simulink model "Sim_main"  (R2025a)
settings: Solver=FixedStepAuto  StartTime=0.0  StopTime=8760  FixedStep=1  RelTol=1e-3
values from neighbouring files (symbols this model uses):
  A = R * 2 * H    [LCOW_calculation.m]    (also in RUN_Simulink_POOL.m; RUN_Simulink_RandomSet.m; RUN_Simulink_SINGLE.m = 12.786871552)
  Cf = 36000    [RUN_Simulink_POOL.m]    (also in RUN_Simulink_RandomSet.m; RUN_Simulink_SINGLE.m)
  CutIn = 3    [RUN_Simulink_POOL.m]    (also in RUN_Simulink_RandomSet.m; RUN_Simulink_SINGLE.m)
  IP1 = (n/(n-1))*P1*( (P2/P1)^((n-1)/n) - 1)    (= 259255.992944)    [RUN_Simulink_POOL.m]    (also in RUN_Simulink_RandomSet.m; RUN_Simulink_SINGLE.m)
  J1 = 1.5 * As    [RUN_Simulink_POOL.m]    (also in RUN_Simulink_RandomSet.m; RUN_Simulink_SINGLE.m = 4.38)
  Limit_Tor = Tor_rq * 0.5    (= 2.3371585434)    [RUN_Simulink_POOL.m]    (also in RUN_Simulink_RandomSet.m; RUN_Simulink_SINGLE.m = 3.45899464424)
  N_PV = data.N_PV(i)    [LCOW_calculation.m]    (also in MOO_Qp_LCOW_CO2.m = optimvar("N_PV","Type","integer","LowerBound",1,"UpperBound"; RUN_Simulink_POOL.m = N_PV_values(i); RUN_Simulink_RandomSet.m = N_PV_values; RUN_Simulink_SINGLE.m = 2)
  N_ro = data.N_ro(i)    [LCOW_calculation.m]    (also in MOO_Qp_LCOW_CO2.m = optimvar("N_ro","Type","integer","LowerBound",2,"UpperBound"; RUN_Simulink_POOL.m = N_ro_values(i); RUN_Simulink_RandomSet.m = N_ro_values; RUN_Simulink_SINGLE.m = 6)
  Nt = data.Nt(i)    [LCOW_calculation.m]    (also in MOO_Qp_LCOW_CO2.m = optimvar("Nt","Type","integer","LowerBound",10,"UpperBound",; RUN_Simulink_POOL.m = Nt_values(i); RUN_Simulink_RandomSet.m = Nt_values; RUN_Simulink_SINGLE.m = 58)
  P2 = 800000    [RUN_Simulink_POOL.m]    (also in RUN_Simulink_RandomSet.m; RUN_Simulink_SINGLE.m)
  R = 0.515 * As    [LCOW_calculation.m]    (also in RUN_Simulink_POOL.m; RUN_Simulink_RandomSet.m; RUN_Simulink_SINGLE.m = 1.5038)
  Tor_rq = IP1 * Va * 10 / (17 * pi)    (= 4.67431708681)    [RUN_Simulink_POOL.m]    (also in RUN_Simulink_RandomSet.m; RUN_Simulink_SINGLE.m = 6.91798928848)
  TR = data.TR(i)    [LCOW_calculation.m]    (also in MOO_Qp_LCOW_CO2.m = optimvar("TR","LowerBound",3,"UpperBound",10); RUN_Simulink_POOL.m = TR_values(i); RUN_Simulink_RandomSet.m = TR_values; RUN_Simulink_SINGLE.m = 9.36)
  Va = e_vol * Vs    (= 9.6291546017e-05)    [RUN_Simulink_POOL.m]    (also in RUN_Simulink_RandomSet.m; RUN_Simulink_SINGLE.m = 0.000142511488105)
  Vf1 = ((P1+Pa)*T2/(T1*(P2+Pa)))*1000    (= 339.891157105)    [RUN_Simulink_POOL.m]    (also in RUN_Simulink_RandomSet.m; RUN_Simulink_SINGLE.m)
  Vt = 2000    [RUN_Simulink_POOL.m]    (also in RUN_Simulink_RandomSet.m; RUN_Simulink_SINGLE.m)
undefined symbols (not defined in the file or in its folder): magnitude
libraries: statsLibrary x36, simulink x1
(part 3 of 4)

== system Sim_main/Transmission ==
  note: Transmission ratios and lossws on the system
  note: Q_pump = Q_rotor (1- losses_trans )*i
  note: W_pump = W_rotor*i
  note: Transmission ratios of rotaional speed
  W_rotor : Inport
  Torque : Inport  Port=2
  Divide : Product  Inputs=/*  RndMeth=Zero  SaturateOnIntegerOverflow=on
  Product : Product
  losses_trans : Gain  Gain=1-0.12
  trans_ratio : Constant  Value=TR
  trans_ratio1 : Constant  Value=TR
  W_Trans : Outport
  Q_trans : Outport  Port=2
  wires:
  trans_ratio1/1 -> Divide/1
  Divide/1 -> losses_trans/1
  losses_trans/1 -> Q_trans/1
  W_rotor/1 -> Product/2
  Torque/1 -> Divide/2
  trans_ratio/1 -> Product/1
  Product/1 -> W_Trans/1

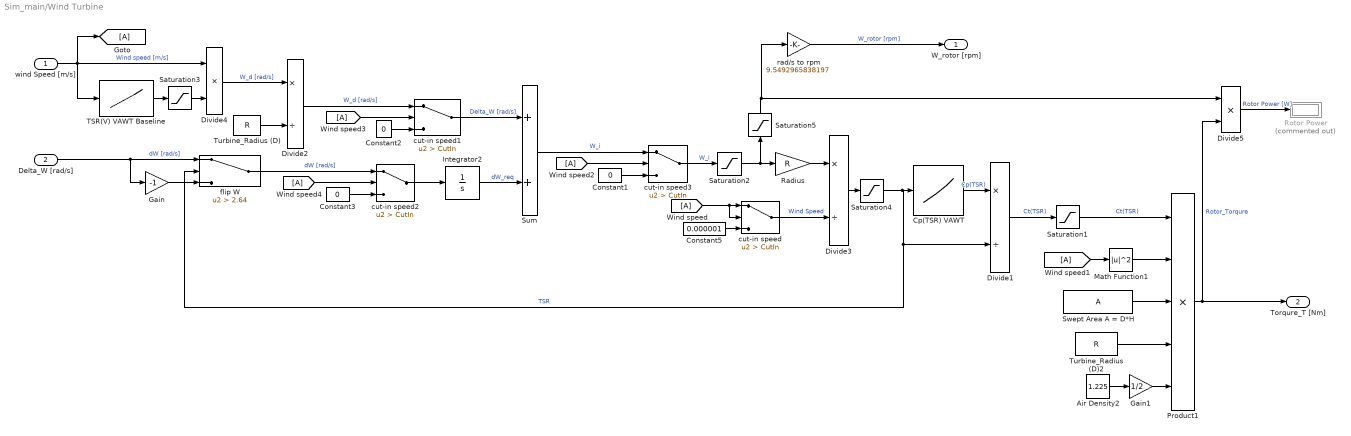
== system Sim_main/Wind Turbine ==
  wind Speed [m/s] : Inport
  Delta_W [rad/s] : Inport  Port=2
  Air Density2 : Constant  Value=1.225
  Constant1 : Constant  Value=0
  Constant2 : Constant  Value=0
  Constant3 : Constant  Value=0
  Constant5 : Constant  Value=0.000001
  Cp(TSR) VAWT : Lookup_n-D  NumberOfTableDimensions=1  BreakpointsForDimension1=[1.439502;1.679111;2.035892;2.329388;2.509915;2.636906;3.080976;3.291367]  Table=[0.01305;0.045283;0.137264;0.259906;0.301179;0.312972;0.285063;0.25283]  InternalRulePriority=Speed  RndMeth=Simplest
  Divide1 : Product  Inputs=*/
  Divide2 : Product  Inputs=*/
  Divide3 : Product  Inputs=*/
  Divide4 : Product  Inputs=**
  Divide5 : Product  Inputs=**
  Gain : Gain  Gain=-1
  Gain1 : Gain  Gain=1/2
  Goto : Goto
  Integrator2 : Integrator  LowerSaturationLimit=-3
  Math Function1 : Math  Operator=magnitude^2
  Product1 : Product  Inputs=5
  Radius : Gain  Gain=R
  Rotor Power : Display  Commented=on
  Saturation1 : Saturate  UpperLimit=inf  LowerLimit=0
  Saturation2 : Saturate  UpperLimit=inf  LowerLimit=0
  Saturation3 : Saturate  UpperLimit=inf  LowerLimit=0.000001
  Saturation4 : Saturate  UpperLimit=6  LowerLimit=0.000001
  Saturation5 : Saturate  UpperLimit=inf  LowerLimit=0.000001
  Sum : Sum
  Swept Area A = D*H : Constant  Value=A
  TSR(V) VAWT Baseline : Lookup_n-D  NumberOfTableDimensions=1  BreakpointsForDimension1=[1;2;4;6;8;10;12]  Table=[0;1;2.4;2.85;3.57;3.96;4.22]  InternalRulePriority=Speed  RndMeth=Simplest
  Turbine_Radius (D) : Constant  Value=R
  Turbine_Radius (D)2 : Constant  Value=R
  Wind speed{,1..4} (5 alike) : From
  cut-in speed{,1..3} (4 alike) : Switch  Criteria=u2 > Threshold  Threshold=CutIn  SaturateOnIntegerOverflow=off  InputSameDT=off
  flip W : Switch  Criteria=u2 > Threshold  Threshold=2.64  SaturateOnIntegerOverflow=off  InputSameDT=off
  rad/s to rpm : Gain  Gain=9.5492965838197
  W_rotor [rpm] : Outport
  Torqure_T [Nm] : Outport  Port=2
  wires:
  wind Speed [m/s]/1 -> Goto/1, TSR(V) VAWT Baseline/1, Divide4/1  "Wind speed [m/s]"
  Divide5/1 -> Rotor Power/1  "Rotor Power [W]"
  Wind speed4/1 -> cut-in speed2/2
  Divide4/1 -> Divide2/1  "W_d [rad/s]"
  Saturation3/1 -> Divide4/2
  TSR(V) VAWT Baseline/1 -> Saturation3/1
  Sum/1 -> cut-in speed3/1  "W_i"
  Wind speed2/1 -> cut-in speed3/2
  Constant1/1 -> cut-in speed3/3
  cut-in speed2/1 -> Integrator2/1
  cut-in speed/1 -> Divide3/2  "Wind Speed"
  Constant5/1 -> cut-in speed/3
  Wind speed/1 -> cut-in speed/2, cut-in speed/1
  Constant3/1 -> cut-in speed2/3
  cut-in speed1/1 -> Sum/1  "Delta_W [rad/s]"
  Constant2/1 -> cut-in speed1/3
  Wind speed3/1 -> cut-in speed1/2
  rad/s to rpm/1 -> W_rotor [rpm]/1  "W_rotor [rpm]"
  Saturation1/1 -> Product1/1  "Ct(TSR)"
  Cp(TSR) VAWT/1 -> Divide1/1  "Cp(TSR)"
  Gain1/1 -> Product1/5
  Divide2/1 -> cut-in speed1/1  "W_d [rad/s]"
  Product1/1 -> Torqure_T [Nm]/1, Divide5/2  "Rotor_Torqure"
  Turbine_Radius (D)2/1 -> Product1/4
  Swept Area A = D*H/1 -> Product1/3
  Wind speed1/1 -> Math Function1/1
  Math Function1/1 -> Product1/2
  Air Density2/1 -> Gain1/1
  Divide1/1 -> Saturation1/1  "Ct(TSR)"
  Divide3/1 -> Saturation4/1
  Radius/1 -> Divide3/1
  Turbine_Radius (D)/1 -> Divide2/2
  cut-in speed3/1 -> Saturation2/1  "W_i"
  Saturation2/1 -> Saturation5/1, Radius/1
  Saturation5/1 -> rad/s to rpm/1, Divide5/1
  Integrator2/1 -> Sum/2  "dW_req"
  flip W/1 -> cut-in speed2/1  "dW [rad/s]"
  Gain/1 -> flip W/3
  Delta_W [rad/s]/1 -> Gain/1, flip W/1  "dW [rad/s]"
  Saturation4/1 -> flip W/2, Divide1/2, Cp(TSR) VAWT/1  "TSR"

== system Sim_main/Pumps/Air operated pump ==
  Air_in : Inport
  P_in : Inport  Port=2
  Air [l/s] to water buckup1 : Lookup_n-D  BreakpointsForDimension1=[1;4;6;8;10;12;14]  BreakpointsForDimension2=[4.8 6.8 8.3]  Table=[6.4 4.22 3.7;28.27 20.5 17.54;44.82 32.5 27.24;63.58 45.5 34.6;86.46 59.3 49;86.46 75.2 61.37;86.46 93 73.8]  InternalRulePriority=Speed  RndMeth=Simplest
      settings: InputPortMap=u0,u1
  Gain1 : Gain  Gain=1/3600
  Saturation : Saturate  UpperLimit=inf  LowerLimit=0
  Saturation2 : Saturate  UpperLimit=inf  LowerLimit=0
  buckup1 : Lookup_n-D  BreakpointsForDimension1=[1;2.76;4.52;6.28;8.04;9.8;11.56;13.32;15.08;16.84;18.6;20.36;22.12;23.88;25.64;27.4;29.16;30.92;32.68;34.44;36.2;37.96;39.72;41.48;43.24;45;46.76;48.52;50.28;52.04;53.8;55.56;57.32;59.08;60.84;62.6;64.36;66.12;67.88;69.64;71.4;73.16;74.92;76.68;78.44;80.2]  BreakpointsForDimension2=[4.8;6.8;8.3]  Table=[33.96748 49.87303 59.5914;33.76481 49.31838 58.97968;33.48128 48.77087 58.35368;33.14781 48.22336 57.75622;32.88569 47.71152 57.1445;32.55935 47.18541 56.49234;32.26869 46.66644 56.03308;31.94236 46.14746 55.45677;31.65883 45.63562 54.78321;31.32536 45.15232 54.24284;31.02043 44.63335 53.65252;30.7155 44.13578 53.0836;30.39629 43.67389 52.53609;30.0985 43.21199 51.96717;29.76503 42.70015 51.41252;29.46723 42.25966 50.85074;29.14089 41.79063 50.32463;28.81456 41.31446 49.78425;28.50249 40.8597 49.23674;28.15475 40.42634 48.71777;27.84982 39.95731 48.19879;27.53062 39.54536 47.68695;27.21142 39.112 47.17511;26.90649 38.68578 46.65614;26.54448 38.25956 46.1443;26.21814 37.8048 45.64673;25.89181 37.58073 45.14203;25.55834 37.04273 44.673;25.21773 36.65456 44.20397;24.90567 36.26401 43.71353;24.53652 35.8806 43.2231;24.21732 35.45913 42.71601;23.86958 35.11377 42.31357;23.52898 34.7803 41.88735;23.18837 34.41829 41.36124;22.84776 34.05628 40.91362;22.50003 33.69427 40.44459;22.15942 33.3394 40.08258;21.81881 33.00593 39.63495;21.45681 32.62965 39.19446;21.10907 32.36752 38.7611;20.77559 32.02692 38.27542;20.40645 31.70058 37.82304;20.05871 31.38852 37.62751;19.70384 31.07645 37.26074;19.22529 30.84559 36.75502]  InternalRulePriority=Speed  RndMeth=Simplest
      settings: InputPortMap=u0,u1
  l/m to m3/h : Gain  Gain=0.06
  Feed flow m3/h : Outport
  Backpressure [bar] : Outport  Port=2
  wires:
  l/m to m3/h/1 -> Feed flow m3/h/1  "Feed flow m3/h"
  Air [l/s] to water buckup1/1 -> Saturation2/1  "water L/m"
  Air_in/1 -> Gain1/1
  Gain1/1 -> Air [l/s] to water buckup1/1
  P_in/1 -> Air [l/s] to water buckup1/2, buckup1/2
  buckup1/1 -> Saturation/1
  Saturation/1 -> Backpressure [bar]/1
  Saturation2/1 -> buckup1/1, l/m to m3/h/1

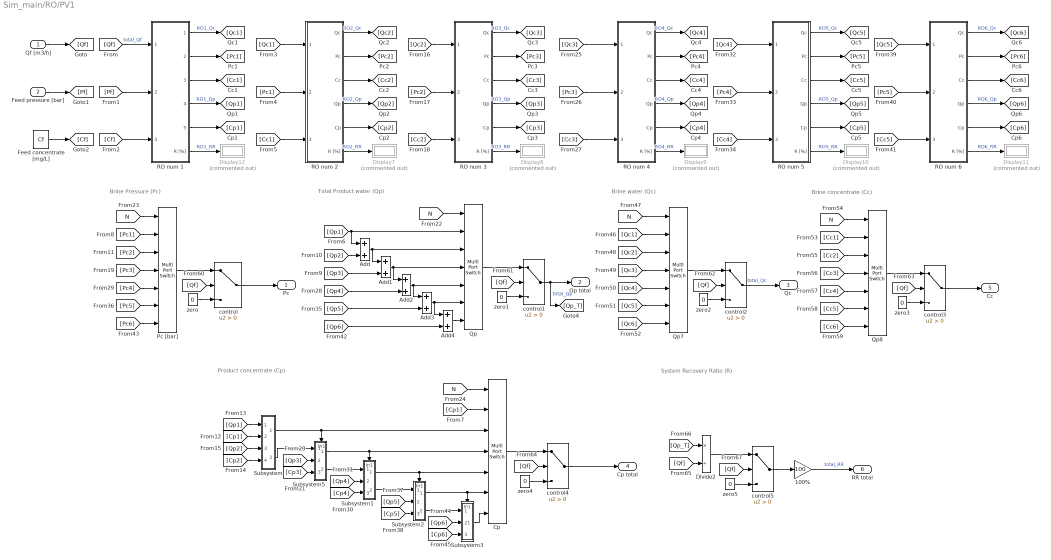
== system Sim_main/RO/PV1 ==
  note: System Recovery Ratio (R)
  note: Brine concentrate (Cc)
  note: Product concentrate (Cp)
  note: Brine water (Qc)
  note: Total Product water (Qp)
  note: Brine Pressure (Pc)
  Qf [m3/h] : Inport
  Feed pressure [bar] : Inport  Port=2
  100% : Gain  Gain=100
  Add{,1..4} (5 alike) : Sum
  Cp : MultiPortSwitch  Inputs=6  SaturateOnIntegerOverflow=off  InputSameDT=off
  Display{7..12} (6 alike) : Display  Commented=on
  Divide2 : Product  Inputs=*/
  Feed concentrate [mg/L] : Constant  Value=Cf
  Pc [bar] : MultiPortSwitch  Inputs=6  SaturateOnIntegerOverflow=off  InputSameDT=off
  Qp : MultiPortSwitch  Inputs=6  SaturateOnIntegerOverflow=off  InputSameDT=off
  Qp7 : MultiPortSwitch  Inputs=6  SaturateOnIntegerOverflow=off  InputSameDT=off
  Qp8 : MultiPortSwitch  Inputs=6  SaturateOnIntegerOverflow=off  InputSameDT=off
  RO num 1 : Subsystem
  RO num 2 : Subsystem
  RO num 3 : Subsystem
  RO num 4 : Subsystem
  RO num 5 : Subsystem
  RO num 6 : Subsystem
  Subsystem : Subsystem
  Subsystem1 : Subsystem
      settings: PortSchema="{\"entries\":[{\"content\":{\"sides\":[{\"content\":{\"connectorIds\":[\"In1\",\"In2\",\"In3\"]},\"type\":\"ConnectorPlacement.EquallySpacedRectSide\",\"uuid\":\"d5ba013f-6078-4f30-8328-72ed2cb8129b\"},{\"content\":{\"connectorIds\":[\"Out1\",\"Out2\"],\"side\":\"RIGHT\"},\"type\":\"ConnectorPlacement.EquallySpacedRectSide\",\"uuid\":\"ed7cb065-416c-47c0-a617-1717dea4ab53\"},{\"content\":{\"connectorIds\":[\"In4\"],\"side\":\"TOP\"},\"type\":\"ConnectorPlacement.EquallySpacedRectSide\",\"uuid\":\"ec2d37e4-f712-4138-a382-b2b31ae58dd4\"}]},\"type\":\"ConnectorPlacement.EquallySpacedConnector\",\"uuid\":\"e33a2c60-ddf6-4c9a-9e3a-37228ac662ce\"}],\"packageUris\":[\"http://schema.mathworks.com/mf0/Connector/R2020b\"],\"version\":\"1.0\"}"
  Subsystem2 : Subsystem
      settings: PortSchema="{\"entries\":[{\"content\":{\"sides\":[{\"content\":{\"connectorIds\":[\"In1\",\"In2\",\"In3\"]},\"type\":\"ConnectorPlacement.EquallySpacedRectSide\",\"uuid\":\"d5ba013f-6078-4f30-8328-72ed2cb8129b\"},{\"content\":{\"connectorIds\":[\"Out1\",\"Out2\"],\"side\":\"RIGHT\"},\"type\":\"ConnectorPlacement.EquallySpacedRectSide\",\"uuid\":\"ed7cb065-416c-47c0-a617-1717dea4ab53\"},{\"content\":{\"connectorIds\":[\"In4\"],\"side\":\"TOP\"},\"type\":\"ConnectorPlacement.EquallySpacedRectSide\",\"uuid\":\"ec2d37e4-f712-4138-a382-b2b31ae58dd4\"}]},\"type\":\"ConnectorPlacement.EquallySpacedConnector\",\"uuid\":\"e33a2c60-ddf6-4c9a-9e3a-37228ac662ce\"}],\"packageUris\":[\"http://schema.mathworks.com/mf0/Connector/R2020b\"],\"version\":\"1.0\"}"
  Subsystem3 : Subsystem
      settings: PortSchema="{\"entries\":[{\"content\":{\"sides\":[{\"content\":{\"connectorIds\":[\"In1\",\"In2\",\"In3\"]},\"type\":\"ConnectorPlacement.EquallySpacedRectSide\",\"uuid\":\"d5ba013f-6078-4f30-8328-72ed2cb8129b\"},{\"content\":{\"connectorIds\":[\"Out1\"],\"side\":\"RIGHT\"},\"type\":\"ConnectorPlacement.EquallySpacedRectSide\",\"uuid\":\"ed7cb065-416c-47c0-a617-1717dea4ab53\"},{\"content\":{\"connectorIds\":[\"In4\"],\"side\":\"TOP\"},\"type\":\"ConnectorPlacement.EquallySpacedRectSide\",\"uuid\":\"ec2d37e4-f712-4138-a382-b2b31ae58dd4\"}]},\"type\":\"ConnectorPlacement.EquallySpacedConnector\",\"uuid\":\"e33a2c60-ddf6-4c9a-9e3a-37228ac662ce\"}],\"packageUris\":[\"http://schema.mathworks.com/mf0/Connector/R2020b\"],\"version\":\"1.0\"}"
  Subsystem5 : Subsystem
      settings: PortSchema="{\"entries\":[{\"content\":{\"sides\":[{\"content\":{\"connectorIds\":[\"In1\",\"In2\",\"In3\"]},\"type\":\"ConnectorPlacement.EquallySpacedRectSide\",\"uuid\":\"d5ba013f-6078-4f30-8328-72ed2cb8129b\"},{\"content\":{\"connectorIds\":[\"Out1\",\"Out2\"],\"side\":\"RIGHT\"},\"type\":\"ConnectorPlacement.EquallySpacedRectSide\",\"uuid\":\"ed7cb065-416c-47c0-a617-1717dea4ab53\"},{\"content\":{\"connectorIds\":[\"In4\"],\"side\":\"TOP\"},\"type\":\"ConnectorPlacement.EquallySpacedRectSide\",\"uuid\":\"ec2d37e4-f712-4138-a382-b2b31ae58dd4\"}]},\"type\":\"ConnectorPlacement.EquallySpacedConnector\",\"uuid\":\"e33a2c60-ddf6-4c9a-9e3a-37228ac662ce\"}],\"packageUris\":[\"http://schema.mathworks.com/mf0/Connector/R2020b\"],\"version\":\"1.0\"}"
  control{,1..5} (6 alike) : Switch  Criteria=u2 > Threshold  ZeroCross=off  SaturateOnIntegerOverflow=off  InputSameDT=off
  zero{,1..5} (6 alike) : Constant  Value=0
  Pc : Outport
  Qp total : Outport  Port=2
  Qc : Outport  Port=3
  Cp total : Outport  Port=4
  Cc : Outport  Port=5
  RR total : Outport  Port=6
  wires:
  RO num 1/6(R [%]) -> Display12/1  "RO1_RR"
  Add3/1 -> Add4/1, Qp/6
  [Cp1] -> Subsystem/2(In2)
  [Qp4] -> Add2/2
  RO num 5/1(Qc) -> [Qc5]  "RO5_Qc"
  Subsystem/2(Out2) -> Subsystem5/1(In2)
  [Qp4] -> Subsystem1/2(In3)
  RO num 6/5(Cp) -> [Cp6]
  [Pc1] -> Pc [bar]/2
  zero/1 -> control/3
  Subsystem3/1(Out1) -> Cp/7
  [Cc1] -> Qp8/2
  Qp7/1 -> control2/1
  [Qp2] -> Add/2
  [Pf] -> RO num 1/2(Pf [bar])
  [Qc4] -> RO num 5/1(Qf [m3/h])
  Add/1 -> Qp/3, Add1/1
  control1/1 -> Qp total/1, [Qp_T]  "total_Qp"
  RO num 4/2(Pc) -> [Pc4]
  Qf [m3/h]/1 -> [Qf]
  [Cc2] -> Qp8/3
  Qp/1 -> control1/1
  RO num 3/4(Qp) -> [Qp3]  "RO3_Qp"
  [Cp4] -> Subsystem1/3(In4)
  [Pc2] -> RO num 3/2(Pf [bar])
  [Cc5] -> RO num 6/3(Cf [mg/L])
  RO num 6/6(R [%]) -> Display11/1  "RO6_RR"
  [Qp2] -> Subsystem/3(In3)
  [Qc5] -> Qp7/6
  [N] -> Qp8/1
  [Qf] -> control4/2
  RO num 5/6(R [%]) -> Display10/1  "RO5_RR"
  [Qp3] -> Add1/2
  [Qp1] -> Add/1, Qp/2
  RO num 2/3(Cc) -> [Cc2]
  Subsystem2/1(Out1) -> Cp/6, Subsystem3/4(In1)
  Add1/1 -> Qp/4, Add2/1
  RO num 4/5(Cp) -> [Cp4]
  RO num 3/2(Pc) -> [Pc3]
  [Pc2] -> Pc [bar]/3
  RO num 5/2(Pc) -> [Pc5]
  [Pc5] -> Pc [bar]/6
  Add4/1 -> Qp/7
  Feed pressure [bar]/1 -> [Pf]
  RO num 3/1(Qc) -> [Qc3]  "RO3_Qc"
  RO num 6/4(Qp) -> [Qp6]  "RO6_Qp"
  RO num 6/2(Pc) -> [Pc6]
  [Qc3] -> Qp7/4
  Subsystem2/2(Out2) -> Subsystem3/1(In2)
  RO num 5/4(Qp) -> [Qp5]  "RO5_Qp"
  [Cp6] -> Subsystem3/3(In4)
  RO num 1/2(Pc [bar]) -> [Pc1]
  [N] -> Qp7/1
  100%/1 -> RR total/1  "total_RR"
  [Qf] -> control2/2
  Cp/1 -> control4/1
  Subsystem/1(Out1) -> Subsystem5/4(In1), Cp/3
  [Qc5] -> RO num 6/1(Qf [m3/h])
  [Qp5] -> Subsystem2/2(In3)
  RO num 4/1(Qc) -> [Qc4]  "RO4_Qc"
  RO num 1/3(TDSc [mg/L]) -> [Cc1]
  RO num 4/3(Cc) -> [Cc4]
  RO num 2/6(R [%]) -> Display7/1  "RO2_RR"
  RO num 4/6(R [%]) -> Display9/1  "RO4_RR"
  Subsystem5/2(Out2) -> Subsystem1/1(In2)
  control2/1 -> Qc/1  "total_Qc"
  RO num 6/1(Qc) -> [Qc6]  "RO6_Qc"
  [Qp1] -> Subsystem/1(In1)
  [Cc6] -> Qp8/7
  [Cf] -> RO num 1/3(TDSf [mg/L])
  [N] -> Cp/1
  [Cc4] -> Qp8/5
  [Pc4] -> Pc [bar]/5
  RO num 2/2(Pc) -> [Pc2]
  [Qp6] -> Subsystem3/2(In3)
  [Qc3] -> RO num 4/1(Qf [m3/h])
  [Qf] -> RO num 1/1(Qf [m3/h])  "total_Qf"
  [N] -> Qp/1
  Subsystem1/1(Out1) -> Subsystem2/4(In1), Cp/5
  Feed concentrate [mg/L]/1 -> [Cf]
  RO num 1/5(TDSp [mg/L]) -> [Cp1]
  RO num 3/3(Cc) -> [Cc3]
  RO num 1/4(Qp [m3/h]) -> [Qp1]  "RO1_Qp"
  control3/1 -> Cc/1
  [Cc2] -> RO num 3/3(Cf [mg/L])
  RO num 3/5(Cp) -> [Cp3]
  zero5/1 -> control5/3
  [Qp5] -> Add3/2
  Subsystem5/1(Out1) -> Subsystem1/4(In1), Cp/4
  RO num 5/5(Cp) -> [Cp5]
  zero3/1 -> control3/3
  [Qf] -> control/2
  RO num 2/4(Qp) -> [Qp2]  "RO2_Qp"
  [Cp2] -> Subsystem/4(In4)
  [Qp_T] -> Divide2/1
  [Qp3] -> Subsystem5/2(In3)
  [Cp1] -> Cp/2
  Pc [bar]/1 -> control/1
  Divide2/1 -> control5/1
  [Qc6] -> Qp7/7
  [Qp6] -> Add4/2
  [Cc5] -> Qp8/6
  zero4/1 -> control4/3
  [Cc3] -> RO num 4/3(Cf [mg/L])
  zero1/1 -> control1/3
  [Pc3] -> Pc [bar]/4
  [Pc6] -> Pc [bar]/7
  RO num 5/3(Cc) -> [Cc5]
  [Cp5] -> Subsystem2/3(In4)
  [Qf] -> control5/2
  control4/1 -> Cp total/1
  RO num 2/1(Qc) -> [Qc2]  "RO2_Qc"
  [Qf] -> control1/2
  [Qf] -> Divide2/2
  [Cp3] -> Subsystem5/3(In4)
  [Qc2] -> RO num 3/1(Qf [m3/h])
  zero2/1 -> control2/3
  [Pc1] -> RO num 2/2(Pf [bar])
  RO num 4/4(Qp) -> [Qp4]  "RO4_Qp"
  [Cc4] -> RO num 5/3(Cf [mg/L])
  [Qc1] -> Qp7/2
  [Pc3] -> RO num 4/2(Pf [bar])
  RO num 3/6(R [%]) -> Display8/1  "RO3_RR"
  RO num 2/5(Cp) -> [Cp2]
  [Qc4] -> Qp7/5
  Qp8/1 -> control3/1
  [Cc1] -> RO num 2/3(Cf [mg/L])
  [Qc2] -> Qp7/3
  control5/1 -> 100%/1
  [Qf] -> control3/2
  [Pc4] -> RO num 5/2(Pf [bar])
  RO num 6/3(Cc) -> [Cc6]
  Subsystem1/2(Out2) -> Subsystem2/1(In2)
  [Qc1] -> RO num 2/1(Qf [m3/h])
  control/1 -> Pc/1
  Add2/1 -> Qp/5, Add3/1
  [Cc3] -> Qp8/4
  [N] -> Pc [bar]/1
  RO num 1/1(Qc [m3/h]) -> [Qc1]  "RO1_Qc"
  [Pc5] -> RO num 6/2(Pf [bar])

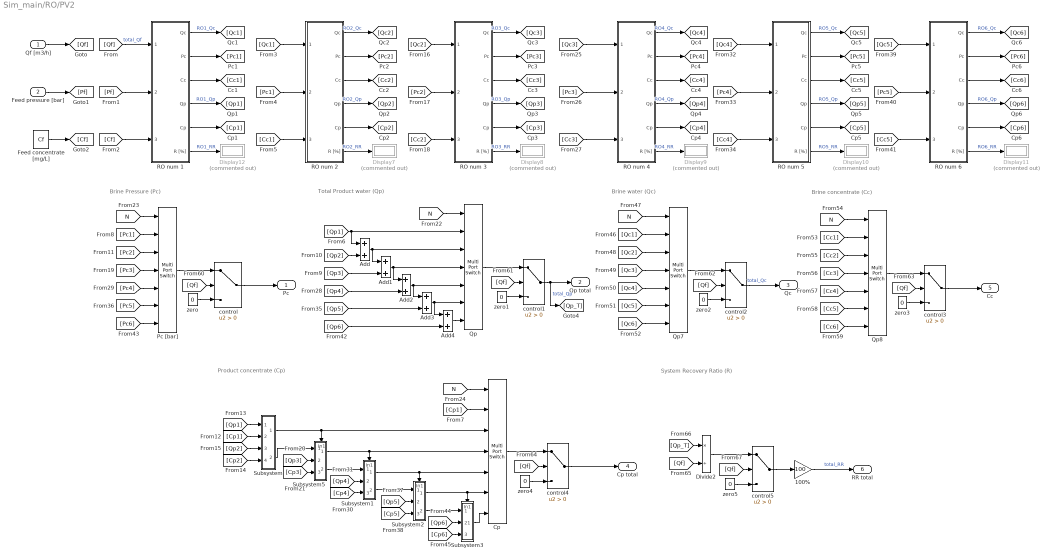
== system Sim_main/RO/PV2 ==
  note: System Recovery Ratio (R)
  note: Brine concentrate (Cc)
  note: Product concentrate (Cp)
  note: Brine water (Qc)
  note: Total Product water (Qp)
  note: Brine Pressure (Pc)
  Qf [m3/h] : Inport
  Feed pressure [bar] : Inport  Port=2
  100% : Gain  Gain=100
  Add{,1..4} (5 alike) : Sum
  Cp : MultiPortSwitch  Inputs=6  SaturateOnIntegerOverflow=off  InputSameDT=off
  Display{7..12} (6 alike) : Display  Commented=on
  Divide2 : Product  Inputs=*/
  Feed concentrate [mg/L] : Constant  Value=Cf
  Pc [bar] : MultiPortSwitch  Inputs=6  SaturateOnIntegerOverflow=off  InputSameDT=off
  Qp : MultiPortSwitch  Inputs=6  SaturateOnIntegerOverflow=off  InputSameDT=off
  Qp7 : MultiPortSwitch  Inputs=6  SaturateOnIntegerOverflow=off  InputSameDT=off
  Qp8 : MultiPortSwitch  Inputs=6  SaturateOnIntegerOverflow=off  InputSameDT=off
  RO num 1 : Subsystem
  RO num 2 : Subsystem
  RO num 3 : Subsystem
  RO num 4 : Subsystem
  RO num 5 : Subsystem
  RO num 6 : Subsystem
  Subsystem : Subsystem
  Subsystem1 : Subsystem
      settings: PortSchema="{\"entries\":[{\"content\":{\"sides\":[{\"content\":{\"connectorIds\":[\"In1\",\"In2\",\"In3\"]},\"type\":\"ConnectorPlacement.EquallySpacedRectSide\",\"uuid\":\"d5ba013f-6078-4f30-8328-72ed2cb8129b\"},{\"content\":{\"connectorIds\":[\"Out1\",\"Out2\"],\"side\":\"RIGHT\"},\"type\":\"ConnectorPlacement.EquallySpacedRectSide\",\"uuid\":\"ed7cb065-416c-47c0-a617-1717dea4ab53\"},{\"content\":{\"connectorIds\":[\"In4\"],\"side\":\"TOP\"},\"type\":\"ConnectorPlacement.EquallySpacedRectSide\",\"uuid\":\"ec2d37e4-f712-4138-a382-b2b31ae58dd4\"}]},\"type\":\"ConnectorPlacement.EquallySpacedConnector\",\"uuid\":\"e33a2c60-ddf6-4c9a-9e3a-37228ac662ce\"}],\"packageUris\":[\"http://schema.mathworks.com/mf0/Connector/R2020b\"],\"version\":\"1.0\"}"
  Subsystem2 : Subsystem
      settings: PortSchema="{\"entries\":[{\"content\":{\"sides\":[{\"content\":{\"connectorIds\":[\"In1\",\"In2\",\"In3\"]},\"type\":\"ConnectorPlacement.EquallySpacedRectSide\",\"uuid\":\"d5ba013f-6078-4f30-8328-72ed2cb8129b\"},{\"content\":{\"connectorIds\":[\"Out1\",\"Out2\"],\"side\":\"RIGHT\"},\"type\":\"ConnectorPlacement.EquallySpacedRectSide\",\"uuid\":\"ed7cb065-416c-47c0-a617-1717dea4ab53\"},{\"content\":{\"connectorIds\":[\"In4\"],\"side\":\"TOP\"},\"type\":\"ConnectorPlacement.EquallySpacedRectSide\",\"uuid\":\"ec2d37e4-f712-4138-a382-b2b31ae58dd4\"}]},\"type\":\"ConnectorPlacement.EquallySpacedConnector\",\"uuid\":\"e33a2c60-ddf6-4c9a-9e3a-37228ac662ce\"}],\"packageUris\":[\"http://schema.mathworks.com/mf0/Connector/R2020b\"],\"version\":\"1.0\"}"
  Subsystem3 : Subsystem
      settings: PortSchema="{\"entries\":[{\"content\":{\"sides\":[{\"content\":{\"connectorIds\":[\"In1\",\"In2\",\"In3\"]},\"type\":\"ConnectorPlacement.EquallySpacedRectSide\",\"uuid\":\"d5ba013f-6078-4f30-8328-72ed2cb8129b\"},{\"content\":{\"connectorIds\":[\"Out1\"],\"side\":\"RIGHT\"},\"type\":\"ConnectorPlacement.EquallySpacedRectSide\",\"uuid\":\"ed7cb065-416c-47c0-a617-1717dea4ab53\"},{\"content\":{\"connectorIds\":[\"In4\"],\"side\":\"TOP\"},\"type\":\"ConnectorPlacement.EquallySpacedRectSide\",\"uuid\":\"ec2d37e4-f712-4138-a382-b2b31ae58dd4\"}]},\"type\":\"ConnectorPlacement.EquallySpacedConnector\",\"uuid\":\"e33a2c60-ddf6-4c9a-9e3a-37228ac662ce\"}],\"packageUris\":[\"http://schema.mathworks.com/mf0/Connector/R2020b\"],\"version\":\"1.0\"}"
  Subsystem5 : Subsystem
      settings: PortSchema="{\"entries\":[{\"content\":{\"sides\":[{\"content\":{\"connectorIds\":[\"In1\",\"In2\",\"In3\"]},\"type\":\"ConnectorPlacement.EquallySpacedRectSide\",\"uuid\":\"d5ba013f-6078-4f30-8328-72ed2cb8129b\"},{\"content\":{\"connectorIds\":[\"Out1\",\"Out2\"],\"side\":\"RIGHT\"},\"type\":\"ConnectorPlacement.EquallySpacedRectSide\",\"uuid\":\"ed7cb065-416c-47c0-a617-1717dea4ab53\"},{\"content\":{\"connectorIds\":[\"In4\"],\"side\":\"TOP\"},\"type\":\"ConnectorPlacement.EquallySpacedRectSide\",\"uuid\":\"ec2d37e4-f712-4138-a382-b2b31ae58dd4\"}]},\"type\":\"ConnectorPlacement.EquallySpacedConnector\",\"uuid\":\"e33a2c60-ddf6-4c9a-9e3a-37228ac662ce\"}],\"packageUris\":[\"http://schema.mathworks.com/mf0/Connector/R2020b\"],\"version\":\"1.0\"}"
  control{,1..5} (6 alike) : Switch  Criteria=u2 > Threshold  ZeroCross=off  SaturateOnIntegerOverflow=off  InputSameDT=off
  zero{,1..5} (6 alike) : Constant  Value=0
  Pc : Outport
  Qp total : Outport  Port=2
  Qc : Outport  Port=3
  Cp total : Outport  Port=4
  Cc : Outport  Port=5
  RR total : Outport  Port=6
  wires:
  RO num 1/6(R [%]) -> Display12/1  "RO1_RR"
  Add3/1 -> Add4/1, Qp/6
  [Cp1] -> Subsystem/2(In2)
  [Qp4] -> Add2/2
  RO num 5/1(Qc) -> [Qc5]  "RO5_Qc"
  Subsystem/2(Out2) -> Subsystem5/1(In2)
  [Qp4] -> Subsystem1/2(In3)
  RO num 6/5(Cp) -> [Cp6]
  [Pc1] -> Pc [bar]/2
  zero/1 -> control/3
  Subsystem3/1(Out1) -> Cp/7
  [Cc1] -> Qp8/2
  Qp7/1 -> control2/1
  [Qp2] -> Add/2
  [Pf] -> RO num 1/2(Pf [bar])
  [Qc4] -> RO num 5/1(Qf [m3/h])
  Add/1 -> Qp/3, Add1/1
  control1/1 -> Qp total/1, [Qp_T]  "total_Qp"
  RO num 4/2(Pc) -> [Pc4]
  Qf [m3/h]/1 -> [Qf]
  [Cc2] -> Qp8/3
  Qp/1 -> control1/1
  RO num 3/4(Qp) -> [Qp3]  "RO3_Qp"
  [Cp4] -> Subsystem1/3(In4)
  [Pc2] -> RO num 3/2(Pf [bar])
  [Cc5] -> RO num 6/3(Cf [mg/L])
  RO num 6/6(R [%]) -> Display11/1  "RO6_RR"
  [Qp2] -> Subsystem/3(In3)
  [Qc5] -> Qp7/6
  [N] -> Qp8/1
  [Qf] -> control4/2
  RO num 5/6(R [%]) -> Display10/1  "RO5_RR"
  [Qp3] -> Add1/2
  [Qp1] -> Add/1, Qp/2
  RO num 2/3(Cc) -> [Cc2]
  Subsystem2/1(Out1) -> Cp/6, Subsystem3/4(In1)
  Add1/1 -> Qp/4, Add2/1
  RO num 4/5(Cp) -> [Cp4]
  RO num 3/2(Pc) -> [Pc3]
  [Pc2] -> Pc [bar]/3
  RO num 5/2(Pc) -> [Pc5]
  [Pc5] -> Pc [bar]/6
  Add4/1 -> Qp/7
  Feed pressure [bar]/1 -> [Pf]
  RO num 3/1(Qc) -> [Qc3]  "RO3_Qc"
  RO num 6/4(Qp) -> [Qp6]  "RO6_Qp"
  RO num 6/2(Pc) -> [Pc6]
  [Qc3] -> Qp7/4
  Subsystem2/2(Out2) -> Subsystem3/1(In2)
  RO num 5/4(Qp) -> [Qp5]  "RO5_Qp"
  [Cp6] -> Subsystem3/3(In4)
  RO num 1/2(Pc) -> [Pc1]
  [N] -> Qp7/1
  100%/1 -> RR total/1  "total_RR"
  [Qf] -> control2/2
  Cp/1 -> control4/1
  Subsystem/1(Out1) -> Subsystem5/4(In1), Cp/3
  [Qc5] -> RO num 6/1(Qf [m3/h])
  [Qp5] -> Subsystem2/2(In3)
  RO num 4/1(Qc) -> [Qc4]  "RO4_Qc"
  RO num 1/3(Cc) -> [Cc1]
  RO num 4/3(Cc) -> [Cc4]
  RO num 2/6(R [%]) -> Display7/1  "RO2_RR"
  RO num 4/6(R [%]) -> Display9/1  "RO4_RR"
  Subsystem5/2(Out2) -> Subsystem1/1(In2)
  control2/1 -> Qc/1  "total_Qc"
  RO num 6/1(Qc) -> [Qc6]  "RO6_Qc"
  [Qp1] -> Subsystem/1(In1)
  [Cc6] -> Qp8/7
  [Cf] -> RO num 1/3(Cf [mg/L])
  [N] -> Cp/1
  [Cc4] -> Qp8/5
  [Pc4] -> Pc [bar]/5
  RO num 2/2(Pc) -> [Pc2]
  [Qp6] -> Subsystem3/2(In3)
  [Qc3] -> RO num 4/1(Qf [m3/h])
  [Qf] -> RO num 1/1(Qf [m3/h])  "total_Qf"
  [N] -> Qp/1
  Subsystem1/1(Out1) -> Subsystem2/4(In1), Cp/5
  Feed concentrate [mg/L]/1 -> [Cf]
  RO num 1/5(Cp) -> [Cp1]
  RO num 3/3(Cc) -> [Cc3]
  RO num 1/4(Qp) -> [Qp1]  "RO1_Qp"
  control3/1 -> Cc/1
  [Cc2] -> RO num 3/3(Cf [mg/L])
  RO num 3/5(Cp) -> [Cp3]
  zero5/1 -> control5/3
  [Qp5] -> Add3/2
  Subsystem5/1(Out1) -> Subsystem1/4(In1), Cp/4
  RO num 5/5(Cp) -> [Cp5]
  zero3/1 -> control3/3
  [Qf] -> control/2
  RO num 2/4(Qp) -> [Qp2]  "RO2_Qp"
  [Cp2] -> Subsystem/4(In4)
  [Qp_T] -> Divide2/1
  [Qp3] -> Subsystem5/2(In3)
  [Cp1] -> Cp/2
  Pc [bar]/1 -> control/1
  Divide2/1 -> control5/1
  [Qc6] -> Qp7/7
  [Qp6] -> Add4/2
  [Cc5] -> Qp8/6
  zero4/1 -> control4/3
  [Cc3] -> RO num 4/3(Cf [mg/L])
  zero1/1 -> control1/3
  [Pc3] -> Pc [bar]/4
  [Pc6] -> Pc [bar]/7
  RO num 5/3(Cc) -> [Cc5]
  [Cp5] -> Subsystem2/3(In4)
  [Qf] -> control5/2
  control4/1 -> Cp total/1
  RO num 2/1(Qc) -> [Qc2]  "RO2_Qc"
  [Qf] -> control1/2
  [Qf] -> Divide2/2
  [Cp3] -> Subsystem5/3(In4)
  [Qc2] -> RO num 3/1(Qf [m3/h])
  zero2/1 -> control2/3
  [Pc1] -> RO num 2/2(Pf [bar])
  RO num 4/4(Qp) -> [Qp4]  "RO4_Qp"
  [Cc4] -> RO num 5/3(Cf [mg/L])
  [Qc1] -> Qp7/2
  [Pc3] -> RO num 4/2(Pf [bar])
  RO num 3/6(R [%]) -> Display8/1  "RO3_RR"
  RO num 2/5(Cp) -> [Cp2]
  [Qc4] -> Qp7/5
  Qp8/1 -> control3/1
  [Cc1] -> RO num 2/3(Cf [mg/L])
  [Qc2] -> Qp7/3
  control5/1 -> 100%/1
  [Qf] -> control3/2
  [Pc4] -> RO num 5/2(Pf [bar])
  RO num 6/3(Cc) -> [Cc6]
  Subsystem1/2(Out2) -> Subsystem2/1(In2)
  [Qc1] -> RO num 2/1(Qf [m3/h])
  control/1 -> Pc/1
  Add2/1 -> Qp/5, Add3/1
  [Cc3] -> Qp8/4
  [N] -> Pc [bar]/1
  RO num 1/1(Qc) -> [Qc1]  "RO1_Qc"
  [Pc5] -> RO num 6/2(Pf [bar])

== system Sim_main/RO/PV1/RO num 1 ==
  note: Recovery ratio (R)
      | $R=Q_p/Q_f$
  note: Concentrate flow rate (Qc)
      | $Qc=Qf-Qp$
  note: Concentrate total dissolved solids (TDSc)
      | $TDS_c=(Q_f*TDS_f-Q_P*TDS_p)/Q_c$
  Qf [m3/h] : Inport
  Pf [bar] : Inport  Port=2
  TDSf [mg/L] : Inport  Port=3
  (Pc) RegressionNeuralNetwork Predict : statsLibrary/Regression/RegressionNeuralNetwork Predict  TrainedLearner=RO_Pc.RegressionNeuralNetwork  OutMin=[]  OutMax=[]  OutputLayerOutMin=[]  OutputLayerOutMax=[]  OutputLayerAdditionOutMin=[]  OutputLayerAdditionOutMax=[]  LayerSelector=Layer 1  Layer1OutMin=[]  Layer1OutMax=[]  Layer1AdditionOutMin=[]  Layer1AdditionOutMax=[]  Layer2OutMin=[]  Layer2OutMax=[]  Layer2AdditionOutMin=[]  Layer2AdditionOutMax=[]  Layer3OutMin=[]  Layer3OutMax=[]  Layer3AdditionOutMin=[]  Layer3AdditionOutMax=[]  Layer4OutMin=[]  Layer4OutMax=[]  Layer4AdditionOutMin=[]  Layer4AdditionOutMax=[]  Layer5OutMin=[]  Layer5OutMax=[]  Layer5AdditionOutMin=[]  Layer5AdditionOutMax=[]  Layer6OutMin=[]  Layer6OutMax=[]  Layer6AdditionOutMin=[]  Layer6AdditionOutMax=[]  Layer7OutMin=[]  Layer7OutMax=[]  Layer7AdditionOutMin=[]  Layer7AdditionOutMax=[]  Layer8OutMin=[]  Layer8OutMax=[]  Layer8AdditionOutMin=[]  Layer8AdditionOutMax=[]  Layer9OutMin=[]  Layer9OutMax=[]  Layer9AdditionOutMin=[]  Layer9AdditionOutMax=[]  Layer10OutMin=[]  Layer10OutMax=[]  Layer10AdditionOutMin=[]  Layer10AdditionOutMax=[]  Layer11OutMin=[]  Layer11OutMax=[]  Layer11AdditionOutMin=[]  Layer11AdditionOutMax=[]  StandardizedInputOutMin=[]  StandardizedInputOutMax=[]  NumHiddenLayers=1
  (Qp) RegressionGP Predict : statsLibrary/Regression/RegressionGP Predict  TrainedLearner=RO_Qp.RegressionGP  ShowOutputSD=off  ShowOutputIntervals=off  Alpha=0.05  OutMin=[]  OutMax=[]  SDOutMin=[]  SDOutMax=[]  IntervalsOutMin=[]  IntervalsOutMax=[]  KernelMin=[]  KernelMax=[]  DistanceOutMin=[]  DistanceOutMax=[]  BasisOutMin=[]  BasisOutMax=[]  StandardizedInputOutMin=[]  StandardizedInputOutMax=[]  KernelParam1Min=[]  KernelParam1Max=[]  KernelParam2Min=[]  KernelParam2Max=[]  KernelParam3Min=[]  KernelParam3Max=[]  KernelParam4Min=[]  KernelParam4Max=[]  BasisParam1Min=[]  BasisParam1Max=[]  BasisParam2Min=[]  BasisParam2Max=[]  SDParam1Min=[]  SDParam1Max=[]  KernelParam5Min=[]  KernelParam5Max=[]
  (TDSp) RegressionNeuralNetwork Predict : statsLibrary/Regression/RegressionNeuralNetwork Predict  TrainedLearner=RO_Cp.RegressionNeuralNetwork  OutMin=[]  OutMax=[]  OutputLayerOutMin=[]  OutputLayerOutMax=[]  OutputLayerAdditionOutMin=[]  OutputLayerAdditionOutMax=[]  LayerSelector=Layer 1  Layer1OutMin=[]  Layer1OutMax=[]  Layer1AdditionOutMin=[]  Layer1AdditionOutMax=[]  Layer2OutMin=[]  Layer2OutMax=[]  Layer2AdditionOutMin=[]  Layer2AdditionOutMax=[]  Layer3OutMin=[]  Layer3OutMax=[]  Layer3AdditionOutMin=[]  Layer3AdditionOutMax=[]  Layer4OutMin=[]  Layer4OutMax=[]  Layer4AdditionOutMin=[]  Layer4AdditionOutMax=[]  Layer5OutMin=[]  Layer5OutMax=[]  Layer5AdditionOutMin=[]  Layer5AdditionOutMax=[]  Layer6OutMin=[]  Layer6OutMax=[]  Layer6AdditionOutMin=[]  Layer6AdditionOutMax=[]  Layer7OutMin=[]  Layer7OutMax=[]  Layer7AdditionOutMin=[]  Layer7AdditionOutMax=[]  Layer8OutMin=[]  Layer8OutMax=[]  Layer8AdditionOutMin=[]  Layer8AdditionOutMax=[]  Layer9OutMin=[]  Layer9OutMax=[]  Layer9AdditionOutMin=[]  Layer9AdditionOutMax=[]  Layer10OutMin=[]  Layer10OutMax=[]  Layer10AdditionOutMin=[]  Layer10AdditionOutMax=[]  Layer11OutMin=[]  Layer11OutMax=[]  Layer11AdditionOutMin=[]  Layer11AdditionOutMax=[]  StandardizedInputOutMin=[]  StandardizedInputOutMax=[]  NumHiddenLayers=1
  100% : Gain  Gain=100
  Divide : Product  Inputs=/*
  Mux : Mux  Inputs=3
  Qf*TDSf : Product
  Qp*TDSp : Product
  Sum : Sum  Inputs=+-
  add2 : Sum  Inputs=+-
  di2 : Product  Inputs=/*
  Qc [m3/h] : Outport
  Pc [bar] : Outport  Port=2
  TDSc [mg/L] : Outport  Port=3
  Qp [m3/h] : Outport  Port=4
  TDSp [mg/L] : Outport  Port=5
  R [%] : Outport  Port=6
  wires:
  (TDSp) RegressionNeuralNetwork Predict/1 -> [TDSp], TDSp [mg/L]/1
  (Pc) RegressionNeuralNetwork Predict/1 -> Pc [bar]/1
  Divide/1 -> 100%/1  "Recovery ratio (R)"
  TDSf [mg/L]/1 -> [TDSf], Mux/3
  Mux/1 -> (Qp) RegressionGP Predict/1, (Pc) RegressionNeuralNetwork Predict/1, (TDSp) RegressionNeuralNetwork Predict/1
  Pf [bar]/1 -> Mux/2
  100%/1 -> R [%]/1
  (Qp) RegressionGP Predict/1 -> Qp [m3/h]/1, [Qp]
  Sum/1 -> di2/1, Qc [m3/h]/1
  [Qf] -> Qf*TDSf/1
  Qf*TDSf/1 -> add2/1
  [Qp] -> Qp*TDSp/1
  [TDSf] -> Qf*TDSf/2
  [TDSp] -> Qp*TDSp/2
  Qp*TDSp/1 -> add2/2
  [Qf] -> Divide/1
  [Qp] -> Divide/2
  [Qf] -> Sum/1
  [Qp] -> Sum/2
  add2/1 -> di2/2
  di2/1 -> TDSc [mg/L]/1
  Qf [m3/h]/1 -> [Qf], Mux/1

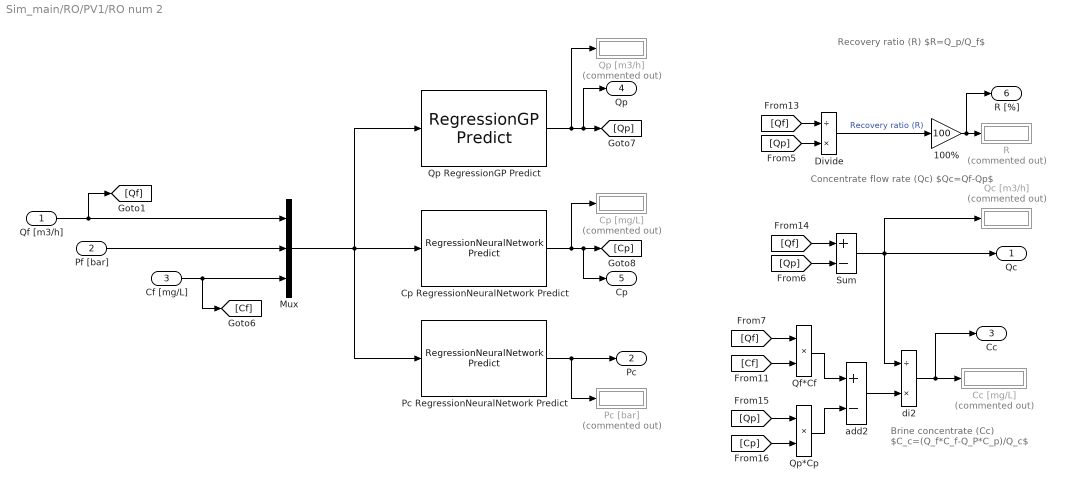
== system Sim_main/RO/PV1/RO num 2 ==
  note: Brine concentrate (Cc)
      | $C_c=(Q_f*C_f-Q_P*C_p)/Q_c$
  note: Concentrate flow rate (Qc)
      | $Qc=Qf-Qp$
  note: Recovery ratio (R)
      | $R=Q_p/Q_f$
  Qf [m3/h] : Inport
  Pf [bar] : Inport  Port=2
  Cf [mg/L] : Inport  Port=3
  100% : Gain  Gain=100
  Cc [mg/L] : Display  Commented=on
      settings: Format=bank
  Cp RegressionNeuralNetwork Predict : statsLibrary/Regression/RegressionNeuralNetwork Predict  TrainedLearner=RO_Cp.RegressionNeuralNetwork  OutMin=[]  OutMax=[]  OutputLayerOutMin=[]  OutputLayerOutMax=[]  OutputLayerAdditionOutMin=[]  OutputLayerAdditionOutMax=[]  LayerSelector=Layer 1  Layer1OutMin=[]  Layer1OutMax=[]  Layer1AdditionOutMin=[]  Layer1AdditionOutMax=[]  Layer2OutMin=[]  Layer2OutMax=[]  Layer2AdditionOutMin=[]  Layer2AdditionOutMax=[]  Layer3OutMin=[]  Layer3OutMax=[]  Layer3AdditionOutMin=[]  Layer3AdditionOutMax=[]  Layer4OutMin=[]  Layer4OutMax=[]  Layer4AdditionOutMin=[]  Layer4AdditionOutMax=[]  Layer5OutMin=[]  Layer5OutMax=[]  Layer5AdditionOutMin=[]  Layer5AdditionOutMax=[]  Layer6OutMin=[]  Layer6OutMax=[]  Layer6AdditionOutMin=[]  Layer6AdditionOutMax=[]  Layer7OutMin=[]  Layer7OutMax=[]  Layer7AdditionOutMin=[]  Layer7AdditionOutMax=[]  Layer8OutMin=[]  Layer8OutMax=[]  Layer8AdditionOutMin=[]  Layer8AdditionOutMax=[]  Layer9OutMin=[]  Layer9OutMax=[]  Layer9AdditionOutMin=[]  Layer9AdditionOutMax=[]  Layer10OutMin=[]  Layer10OutMax=[]  Layer10AdditionOutMin=[]  Layer10AdditionOutMax=[]  Layer11OutMin=[]  Layer11OutMax=[]  Layer11AdditionOutMin=[]  Layer11AdditionOutMax=[]  StandardizedInputOutMin=[]  StandardizedInputOutMax=[]  NumHiddenLayers=1
  Cp [mg/L] : Display  Commented=on
  Divide : Product  Inputs=/*
  Mux : Mux  Inputs=3
  Pc RegressionNeuralNetwork Predict : statsLibrary/Regression/RegressionNeuralNetwork Predict  TrainedLearner=RO_Pc.RegressionNeuralNetwork  OutMin=[]  OutMax=[]  OutputLayerOutMin=[]  OutputLayerOutMax=[]  OutputLayerAdditionOutMin=[]  OutputLayerAdditionOutMax=[]  LayerSelector=Layer 1  Layer1OutMin=[]  Layer1OutMax=[]  Layer1AdditionOutMin=[]  Layer1AdditionOutMax=[]  Layer2OutMin=[]  Layer2OutMax=[]  Layer2AdditionOutMin=[]  Layer2AdditionOutMax=[]  Layer3OutMin=[]  Layer3OutMax=[]  Layer3AdditionOutMin=[]  Layer3AdditionOutMax=[]  Layer4OutMin=[]  Layer4OutMax=[]  Layer4AdditionOutMin=[]  Layer4AdditionOutMax=[]  Layer5OutMin=[]  Layer5OutMax=[]  Layer5AdditionOutMin=[]  Layer5AdditionOutMax=[]  Layer6OutMin=[]  Layer6OutMax=[]  Layer6AdditionOutMin=[]  Layer6AdditionOutMax=[]  Layer7OutMin=[]  Layer7OutMax=[]  Layer7AdditionOutMin=[]  Layer7AdditionOutMax=[]  Layer8OutMin=[]  Layer8OutMax=[]  Layer8AdditionOutMin=[]  Layer8AdditionOutMax=[]  Layer9OutMin=[]  Layer9OutMax=[]  Layer9AdditionOutMin=[]  Layer9AdditionOutMax=[]  Layer10OutMin=[]  Layer10OutMax=[]  Layer10AdditionOutMin=[]  Layer10AdditionOutMax=[]  Layer11OutMin=[]  Layer11OutMax=[]  Layer11AdditionOutMin=[]  Layer11AdditionOutMax=[]  StandardizedInputOutMin=[]  StandardizedInputOutMax=[]  NumHiddenLayers=1
  Pc [bar] : Display  Commented=on
  Qc [m3/h] : Display  Commented=on
  Qf*Cf : Product
  Qp RegressionGP Predict : statsLibrary/Regression/RegressionGP Predict  TrainedLearner=RO_Qp.RegressionGP  ShowOutputSD=off  ShowOutputIntervals=off  Alpha=0.05  OutMin=[]  OutMax=[]  SDOutMin=[]  SDOutMax=[]  IntervalsOutMin=[]  IntervalsOutMax=[]  KernelMin=[]  KernelMax=[]  DistanceOutMin=[]  DistanceOutMax=[]  BasisOutMin=[]  BasisOutMax=[]  StandardizedInputOutMin=[]  StandardizedInputOutMax=[]  KernelParam1Min=[]  KernelParam1Max=[]  KernelParam2Min=[]  KernelParam2Max=[]  KernelParam3Min=[]  KernelParam3Max=[]  KernelParam4Min=[]  KernelParam4Max=[]  BasisParam1Min=[]  BasisParam1Max=[]  BasisParam2Min=[]  BasisParam2Max=[]  SDParam1Min=[]  SDParam1Max=[]  KernelParam5Min=[]  KernelParam5Max=[]
  Qp [m3/h] : Display  Commented=on
  Qp*Cp : Product
  R : Display  Commented=on
  Sum : Sum  Inputs=+-
  add2 : Sum  Inputs=+-
  di2 : Product  Inputs=/*
  Qc : Outport
  Pc : Outport  Port=2
  Cc : Outport  Port=3
  Qp : Outport  Port=4
  Cp : Outport  Port=5
  R [%] : Outport  Port=6
  wires:
  di2/1 -> Cc [mg/L]/1, Cc/1
  add2/1 -> di2/2
  [Qp] -> Sum/2
  [Qf] -> Sum/1
  [Qp] -> Divide/2
  [Qf] -> Divide/1
  Qp*Cp/1 -> add2/2
  [Cp] -> Qp*Cp/2
  [Cf] -> Qf*Cf/2
  [Qp] -> Qp*Cp/1
  Qf*Cf/1 -> add2/1
  [Qf] -> Qf*Cf/1
  Sum/1 -> Qc [m3/h]/1, Qc/1, di2/1
  Qp RegressionGP Predict/1 -> Qp [m3/h]/1, [Qp], Qp/1
  100%/1 -> R [%]/1, R/1
  Qf [m3/h]/1 -> Mux/1, [Qf]
  Pf [bar]/1 -> Mux/2
  Mux/1 -> Cp RegressionNeuralNetwork Predict/1, Qp RegressionGP Predict/1, Pc RegressionNeuralNetwork Predict/1
  Cf [mg/L]/1 -> [Cf], Mux/3
  Divide/1 -> 100%/1  "Recovery ratio (R)"
  Pc RegressionNeuralNetwork Predict/1 -> Pc [bar]/1, Pc/1
  Cp RegressionNeuralNetwork Predict/1 -> Cp [mg/L]/1, [Cp], Cp/1

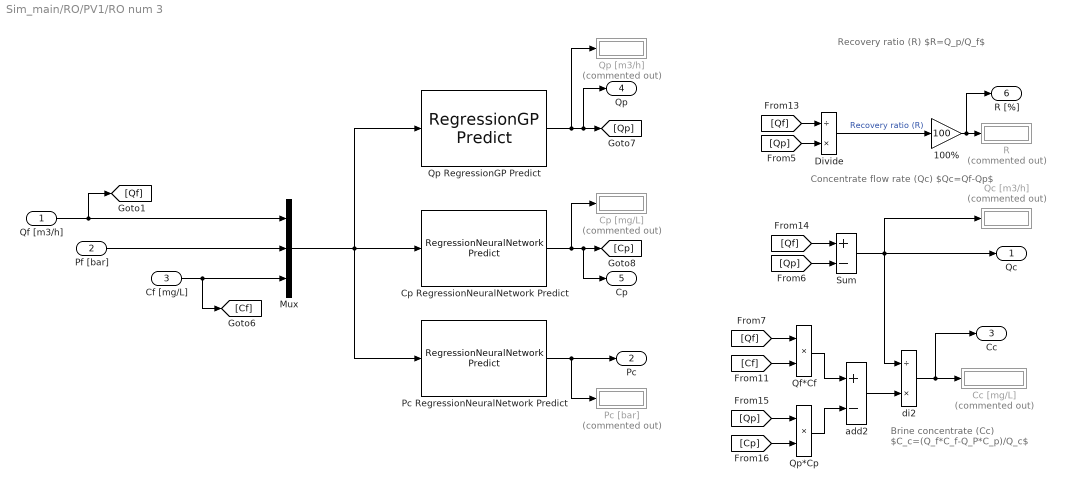
== system Sim_main/RO/PV1/RO num 3 ==
  note: Recovery ratio (R)
      | $R=Q_p/Q_f$
  note: Concentrate flow rate (Qc)
      | $Qc=Qf-Qp$
  note: Brine concentrate (Cc)
      | $C_c=(Q_f*C_f-Q_P*C_p)/Q_c$
  Qf [m3/h] : Inport
  Pf [bar] : Inport  Port=2
  Cf [mg/L] : Inport  Port=3
  100% : Gain  Gain=100
  Cc [mg/L] : Display  Commented=on
      settings: Format=bank
  Cp RegressionNeuralNetwork Predict : statsLibrary/Regression/RegressionNeuralNetwork Predict  TrainedLearner=RO_Cp.RegressionNeuralNetwork  OutMin=[]  OutMax=[]  OutputLayerOutMin=[]  OutputLayerOutMax=[]  OutputLayerAdditionOutMin=[]  OutputLayerAdditionOutMax=[]  LayerSelector=Layer 1  Layer1OutMin=[]  Layer1OutMax=[]  Layer1AdditionOutMin=[]  Layer1AdditionOutMax=[]  Layer2OutMin=[]  Layer2OutMax=[]  Layer2AdditionOutMin=[]  Layer2AdditionOutMax=[]  Layer3OutMin=[]  Layer3OutMax=[]  Layer3AdditionOutMin=[]  Layer3AdditionOutMax=[]  Layer4OutMin=[]  Layer4OutMax=[]  Layer4AdditionOutMin=[]  Layer4AdditionOutMax=[]  Layer5OutMin=[]  Layer5OutMax=[]  Layer5AdditionOutMin=[]  Layer5AdditionOutMax=[]  Layer6OutMin=[]  Layer6OutMax=[]  Layer6AdditionOutMin=[]  Layer6AdditionOutMax=[]  Layer7OutMin=[]  Layer7OutMax=[]  Layer7AdditionOutMin=[]  Layer7AdditionOutMax=[]  Layer8OutMin=[]  Layer8OutMax=[]  Layer8AdditionOutMin=[]  Layer8AdditionOutMax=[]  Layer9OutMin=[]  Layer9OutMax=[]  Layer9AdditionOutMin=[]  Layer9AdditionOutMax=[]  Layer10OutMin=[]  Layer10OutMax=[]  Layer10AdditionOutMin=[]  Layer10AdditionOutMax=[]  Layer11OutMin=[]  Layer11OutMax=[]  Layer11AdditionOutMin=[]  Layer11AdditionOutMax=[]  StandardizedInputOutMin=[]  StandardizedInputOutMax=[]  NumHiddenLayers=1
  Cp [mg/L] : Display  Commented=on
  Divide : Product  Inputs=/*
  Mux : Mux  Inputs=3
  Pc RegressionNeuralNetwork Predict : statsLibrary/Regression/RegressionNeuralNetwork Predict  TrainedLearner=RO_Pc.RegressionNeuralNetwork  OutMin=[]  OutMax=[]  OutputLayerOutMin=[]  OutputLayerOutMax=[]  OutputLayerAdditionOutMin=[]  OutputLayerAdditionOutMax=[]  LayerSelector=Layer 1  Layer1OutMin=[]  Layer1OutMax=[]  Layer1AdditionOutMin=[]  Layer1AdditionOutMax=[]  Layer2OutMin=[]  Layer2OutMax=[]  Layer2AdditionOutMin=[]  Layer2AdditionOutMax=[]  Layer3OutMin=[]  Layer3OutMax=[]  Layer3AdditionOutMin=[]  Layer3AdditionOutMax=[]  Layer4OutMin=[]  Layer4OutMax=[]  Layer4AdditionOutMin=[]  Layer4AdditionOutMax=[]  Layer5OutMin=[]  Layer5OutMax=[]  Layer5AdditionOutMin=[]  Layer5AdditionOutMax=[]  Layer6OutMin=[]  Layer6OutMax=[]  Layer6AdditionOutMin=[]  Layer6AdditionOutMax=[]  Layer7OutMin=[]  Layer7OutMax=[]  Layer7AdditionOutMin=[]  Layer7AdditionOutMax=[]  Layer8OutMin=[]  Layer8OutMax=[]  Layer8AdditionOutMin=[]  Layer8AdditionOutMax=[]  Layer9OutMin=[]  Layer9OutMax=[]  Layer9AdditionOutMin=[]  Layer9AdditionOutMax=[]  Layer10OutMin=[]  Layer10OutMax=[]  Layer10AdditionOutMin=[]  Layer10AdditionOutMax=[]  Layer11OutMin=[]  Layer11OutMax=[]  Layer11AdditionOutMin=[]  Layer11AdditionOutMax=[]  StandardizedInputOutMin=[]  StandardizedInputOutMax=[]  NumHiddenLayers=1
  Pc [bar] : Display  Commented=on
  Qc [m3/h] : Display  Commented=on
  Qf*Cf : Product
  Qp RegressionGP Predict : statsLibrary/Regression/RegressionGP Predict  TrainedLearner=RO_Qp.RegressionGP  ShowOutputSD=off  ShowOutputIntervals=off  Alpha=0.05  OutMin=[]  OutMax=[]  SDOutMin=[]  SDOutMax=[]  IntervalsOutMin=[]  IntervalsOutMax=[]  KernelMin=[]  KernelMax=[]  DistanceOutMin=[]  DistanceOutMax=[]  BasisOutMin=[]  BasisOutMax=[]  StandardizedInputOutMin=[]  StandardizedInputOutMax=[]  KernelParam1Min=[]  KernelParam1Max=[]  KernelParam2Min=[]  KernelParam2Max=[]  KernelParam3Min=[]  KernelParam3Max=[]  KernelParam4Min=[]  KernelParam4Max=[]  BasisParam1Min=[]  BasisParam1Max=[]  BasisParam2Min=[]  BasisParam2Max=[]  SDParam1Min=[]  SDParam1Max=[]  KernelParam5Min=[]  KernelParam5Max=[]
  Qp [m3/h] : Display  Commented=on
  Qp*Cp : Product
  R : Display  Commented=on
  Sum : Sum  Inputs=+-
  add2 : Sum  Inputs=+-
  di2 : Product  Inputs=/*
  Qc : Outport
  Pc : Outport  Port=2
  Cc : Outport  Port=3
  Qp : Outport  Port=4
  Cp : Outport  Port=5
  R [%] : Outport  Port=6
  wires:
  Cp RegressionNeuralNetwork Predict/1 -> Cp/1, [Cp], Cp [mg/L]/1
  Pc RegressionNeuralNetwork Predict/1 -> Pc/1, Pc [bar]/1
  Divide/1 -> 100%/1  "Recovery ratio (R)"
  Cf [mg/L]/1 -> Mux/3, [Cf]
  Mux/1 -> Pc RegressionNeuralNetwork Predict/1, Qp RegressionGP Predict/1, Cp RegressionNeuralNetwork Predict/1
  Pf [bar]/1 -> Mux/2
  Qf [m3/h]/1 -> [Qf], Mux/1
  100%/1 -> R/1, R [%]/1
  Qp RegressionGP Predict/1 -> Qp/1, [Qp], Qp [m3/h]/1
  Sum/1 -> di2/1, Qc/1, Qc [m3/h]/1
  [Qf] -> Qf*Cf/1
  Qf*Cf/1 -> add2/1
  [Qp] -> Qp*Cp/1
  [Cf] -> Qf*Cf/2
  [Cp] -> Qp*Cp/2
  Qp*Cp/1 -> add2/2
  [Qf] -> Divide/1
  [Qp] -> Divide/2
  [Qf] -> Sum/1
  [Qp] -> Sum/2
  add2/1 -> di2/2
  di2/1 -> Cc/1, Cc [mg/L]/1

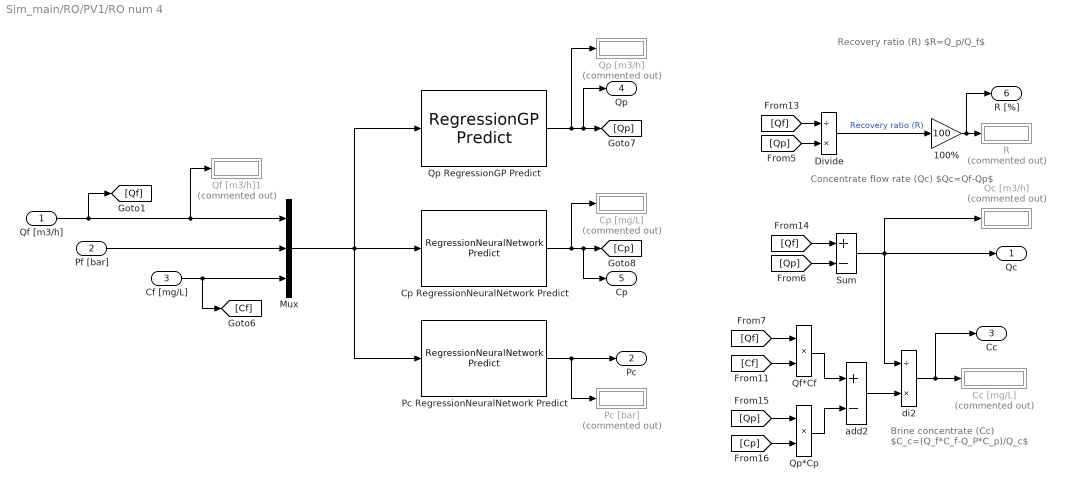
== system Sim_main/RO/PV1/RO num 4 ==
  note: Brine concentrate (Cc)
      | $C_c=(Q_f*C_f-Q_P*C_p)/Q_c$
  note: Concentrate flow rate (Qc)
      | $Qc=Qf-Qp$
  note: Recovery ratio (R)
      | $R=Q_p/Q_f$
  Qf [m3/h] : Inport
  Pf [bar] : Inport  Port=2
  Cf [mg/L] : Inport  Port=3
  100% : Gain  Gain=100
  Cc [mg/L] : Display  Commented=on
      settings: Format=bank
  Cp RegressionNeuralNetwork Predict : statsLibrary/Regression/RegressionNeuralNetwork Predict  TrainedLearner=RO_Cp.RegressionNeuralNetwork  OutMin=[]  OutMax=[]  OutputLayerOutMin=[]  OutputLayerOutMax=[]  OutputLayerAdditionOutMin=[]  OutputLayerAdditionOutMax=[]  LayerSelector=Layer 1  Layer1OutMin=[]  Layer1OutMax=[]  Layer1AdditionOutMin=[]  Layer1AdditionOutMax=[]  Layer2OutMin=[]  Layer2OutMax=[]  Layer2AdditionOutMin=[]  Layer2AdditionOutMax=[]  Layer3OutMin=[]  Layer3OutMax=[]  Layer3AdditionOutMin=[]  Layer3AdditionOutMax=[]  Layer4OutMin=[]  Layer4OutMax=[]  Layer4AdditionOutMin=[]  Layer4AdditionOutMax=[]  Layer5OutMin=[]  Layer5OutMax=[]  Layer5AdditionOutMin=[]  Layer5AdditionOutMax=[]  Layer6OutMin=[]  Layer6OutMax=[]  Layer6AdditionOutMin=[]  Layer6AdditionOutMax=[]  Layer7OutMin=[]  Layer7OutMax=[]  Layer7AdditionOutMin=[]  Layer7AdditionOutMax=[]  Layer8OutMin=[]  Layer8OutMax=[]  Layer8AdditionOutMin=[]  Layer8AdditionOutMax=[]  Layer9OutMin=[]  Layer9OutMax=[]  Layer9AdditionOutMin=[]  Layer9AdditionOutMax=[]  Layer10OutMin=[]  Layer10OutMax=[]  Layer10AdditionOutMin=[]  Layer10AdditionOutMax=[]  Layer11OutMin=[]  Layer11OutMax=[]  Layer11AdditionOutMin=[]  Layer11AdditionOutMax=[]  StandardizedInputOutMin=[]  StandardizedInputOutMax=[]  NumHiddenLayers=1
  Cp [mg/L] : Display  Commented=on
  Divide : Product  Inputs=/*
  Mux : Mux  Inputs=3
  Pc RegressionNeuralNetwork Predict : statsLibrary/Regression/RegressionNeuralNetwork Predict  TrainedLearner=RO_Pc.RegressionNeuralNetwork  OutMin=[]  OutMax=[]  OutputLayerOutMin=[]  OutputLayerOutMax=[]  OutputLayerAdditionOutMin=[]  OutputLayerAdditionOutMax=[]  LayerSelector=Layer 1  Layer1OutMin=[]  Layer1OutMax=[]  Layer1AdditionOutMin=[]  Layer1AdditionOutMax=[]  Layer2OutMin=[]  Layer2OutMax=[]  Layer2AdditionOutMin=[]  Layer2AdditionOutMax=[]  Layer3OutMin=[]  Layer3OutMax=[]  Layer3AdditionOutMin=[]  Layer3AdditionOutMax=[]  Layer4OutMin=[]  Layer4OutMax=[]  Layer4AdditionOutMin=[]  Layer4AdditionOutMax=[]  Layer5OutMin=[]  Layer5OutMax=[]  Layer5AdditionOutMin=[]  Layer5AdditionOutMax=[]  Layer6OutMin=[]  Layer6OutMax=[]  Layer6AdditionOutMin=[]  Layer6AdditionOutMax=[]  Layer7OutMin=[]  Layer7OutMax=[]  Layer7AdditionOutMin=[]  Layer7AdditionOutMax=[]  Layer8OutMin=[]  Layer8OutMax=[]  Layer8AdditionOutMin=[]  Layer8AdditionOutMax=[]  Layer9OutMin=[]  Layer9OutMax=[]  Layer9AdditionOutMin=[]  Layer9AdditionOutMax=[]  Layer10OutMin=[]  Layer10OutMax=[]  Layer10AdditionOutMin=[]  Layer10AdditionOutMax=[]  Layer11OutMin=[]  Layer11OutMax=[]  Layer11AdditionOutMin=[]  Layer11AdditionOutMax=[]  StandardizedInputOutMin=[]  StandardizedInputOutMax=[]  NumHiddenLayers=1
  Pc [bar] : Display  Commented=on
  Qc [m3/h] : Display  Commented=on
  Qf [m3/h]1 : Display  Commented=on
  Qf*Cf : Product
  Qp RegressionGP Predict : statsLibrary/Regression/RegressionGP Predict  TrainedLearner=RO_Qp.RegressionGP  ShowOutputSD=off  ShowOutputIntervals=off  Alpha=0.05  OutMin=[]  OutMax=[]  SDOutMin=[]  SDOutMax=[]  IntervalsOutMin=[]  IntervalsOutMax=[]  KernelMin=[]  KernelMax=[]  DistanceOutMin=[]  DistanceOutMax=[]  BasisOutMin=[]  BasisOutMax=[]  StandardizedInputOutMin=[]  StandardizedInputOutMax=[]  KernelParam1Min=[]  KernelParam1Max=[]  KernelParam2Min=[]  KernelParam2Max=[]  KernelParam3Min=[]  KernelParam3Max=[]  KernelParam4Min=[]  KernelParam4Max=[]  BasisParam1Min=[]  BasisParam1Max=[]  BasisParam2Min=[]  BasisParam2Max=[]  SDParam1Min=[]  SDParam1Max=[]  KernelParam5Min=[]  KernelParam5Max=[]
  Qp [m3/h] : Display  Commented=on
  Qp*Cp : Product
  R : Display  Commented=on
  Sum : Sum  Inputs=+-
  add2 : Sum  Inputs=+-
  di2 : Product  Inputs=/*
  Qc : Outport
  Pc : Outport  Port=2
  Cc : Outport  Port=3
  Qp : Outport  Port=4
  Cp : Outport  Port=5
  R [%] : Outport  Port=6
  wires:
  di2/1 -> Cc [mg/L]/1, Cc/1
  add2/1 -> di2/2
  [Qp] -> Sum/2
  [Qf] -> Sum/1
  [Qp] -> Divide/2
  [Qf] -> Divide/1
  Qp*Cp/1 -> add2/2
  [Cp] -> Qp*Cp/2
  [Cf] -> Qf*Cf/2
  [Qp] -> Qp*Cp/1
  Qf*Cf/1 -> add2/1
  [Qf] -> Qf*Cf/1
  Sum/1 -> Qc [m3/h]/1, Qc/1, di2/1
  Qp RegressionGP Predict/1 -> Qp [m3/h]/1, [Qp], Qp/1
  100%/1 -> R [%]/1, R/1
  Qf [m3/h]/1 -> Qf [m3/h]1/1, Mux/1, [Qf]
  Pf [bar]/1 -> Mux/2
  Mux/1 -> Cp RegressionNeuralNetwork Predict/1, Qp RegressionGP Predict/1, Pc RegressionNeuralNetwork Predict/1
  Cf [mg/L]/1 -> [Cf], Mux/3
  Divide/1 -> 100%/1  "Recovery ratio (R)"
  Pc RegressionNeuralNetwork Predict/1 -> Pc [bar]/1, Pc/1
  Cp RegressionNeuralNetwork Predict/1 -> Cp [mg/L]/1, [Cp], Cp/1
